simulink model "matlab_comm_test"  (R2019a)
settings: Solver=VariableStepAuto  StartTime=0.0  StopTime=inf  RelTol=1e-3
libraries: dspnetwork x2
settings Model: Creator=USRG-ASUS  LastModifiedBy=USRG-ASUS

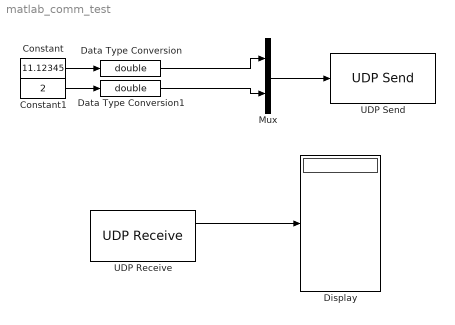
== system matlab_comm_test ==
  Constant : Constant  Value=11.12345
  Constant1 : Constant  Value=2
  Data Type Conversion : DataTypeConversion  OutDataTypeStr=double
  Data Type Conversion1 : DataTypeConversion  OutDataTypeStr=double
  Display : Display
  Mux : Mux  Inputs=2
  UDP Receive : dspnetwork/UDP Receive  localURL='0.0.0.0'  localPort=9090  remoteURL='127.0.0.1'  remotePort=-1  recvBufferSize=40  dims=5  signalDatatype=double  isComplex=off  isVarSize=off  showBlockingTime=off  blockingTime=0  sampletime=-1  blockPlatform=[]
      settings: SourceProductName=Simulink
  UDP Send : dspnetwork/UDP Send  remoteURL='127.0.0.1'  remotePort=8080  localURL='0.0.0.0'  localPortSource=Automatically determine  localPort=-1  sampletime=-1  blockPlatform=[]  separateLengthPort=0
      settings: SourceProductName=Simulink
  wires:
  Constant1/1 -> Data Type Conversion1/1
  Data Type Conversion1/1 -> Mux/2
  Data Type Conversion/1 -> Mux/1
  Mux/1 -> UDP Send/1
  Constant/1 -> Data Type Conversion/1
  UDP Receive/1 -> Display/1
